simulink model "inverse_kinematics_calculator"  (R2019b)
settings: Solver=VariableStepAuto  StartTime=0.0  StopTime=4  RelTol=1e-3
libraries: simulink x3, robotcorelib x1, robotmaniplib x1
settings Model: Creator=PC  LastModifiedBy=PC

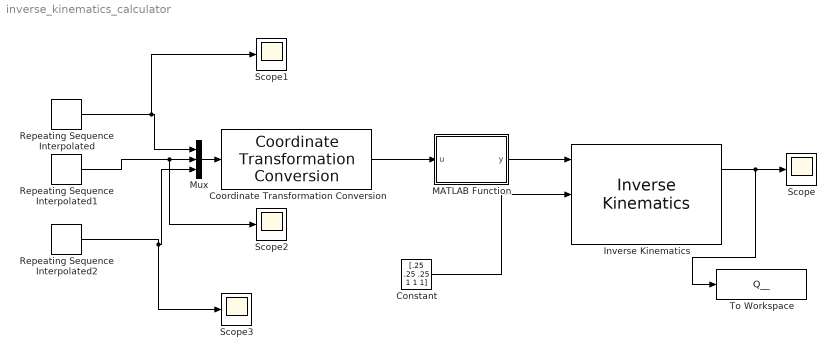
== system inverse_kinematics_calculator ==
  Constant : Constant  Value=[.25 .25 .25 1 1 1]
  Coordinate Transformation Conversion : robotcorelib/Coordinate Transformation Conversion  InputRepresentation=Translation Vector  InputEulerSequence=ZYX  ShowTrVecInputPort=on  OutputRepresentation=Homogeneous Transformation  OutputEulerSequence=ZYX  ShowTrVecOutputPort=on  SimulateUsing=Interpreted execution
      settings: SourceProductBaseCode=RO
  Inverse Kinematics : robotmaniplib/Inverse Kinematics  RigidBodyTree=robot  EndEffector=iiwa_link_ee_kuka  ShowInfo=on  SolverName=BFGS Gradient Projection  EnforceJointLimits=off  MaxIterations=1500  MaxTime=100  GradientTolerance=1e-7  SolutionTolerance=1e-6  StepTolerance=1e-14  ErrorChangeTolerance=1e-12  UseErrorDamping=on  DampingBias=0.0025  SimulateUsing=Interpreted execution
      settings: SourceProductName=Robotics System Toolbox
  MATLAB Function : MATLAB Function  TreatAsAtomicUnit=on
  Mux : Mux  Inputs=3
  Repeating Sequence Interpolated : simulink/Sources/Repeating Sequence Interpolated  OutValues=x  TimeValues=[0 1 2 3]  LookUpMeth=Interpolation-Use End Values  tsamp=1  OutMin=[]  OutMax=[]  OutDataTypeStr=double  OutputDataTypeScalingMode=double  OutDataType=fixdt(0,8)  OutScaling=2^-10
  Repeating Sequence Interpolated1 : simulink/Sources/Repeating Sequence Interpolated  OutValues=y  TimeValues=[0 1 2 3]  LookUpMeth=Interpolation-Use End Values  tsamp=1  OutMin=[]  OutMax=[]  OutDataTypeStr=double  OutputDataTypeScalingMode=double  OutDataType=fixdt(0,8)  OutScaling=2^-10
  Repeating Sequence Interpolated2 : simulink/Sources/Repeating Sequence Interpolated  OutValues=z  TimeValues=[0 1 2 3]  LookUpMeth=Interpolation-Use End Values  tsamp=1  OutMin=[]  OutMax=[]  OutDataTypeStr=double  OutputDataTypeScalingMode=double  OutDataType=fixdt(0,8)  OutScaling=2^-10
  Scope{,1..3} (4 alike) : Scope
  To Workspace : ToWorkspace  VariableName=Q__  SaveFormat=Timeseries  SampleTime=1
  wires:
  Repeating Sequence Interpolated/1 -> Scope1/1, Mux/1
  Repeating Sequence Interpolated1/1 -> Scope2/1, Mux/2
  Repeating Sequence Interpolated2/1 -> Scope3/1, Mux/3
  Mux/1 -> Coordinate Transformation Conversion/1
  Coordinate Transformation Conversion/1 -> MATLAB Function/1(u)
  Constant/1 -> Inverse Kinematics/2
  Inverse Kinematics/1 -> To Workspace/1, Scope/1
  MATLAB Function/1(y) -> Inverse Kinematics/1

== matlab function inverse_kinematics_calculator/MATLAB Function ==
  data: u input; y output
function y = fcn(u)
u(1:3,1:3) = [0 0 0; 0 0 0; 0 0 0];
u(1,3) = -1; 
u(2,2) = 1; 
u(3,1) = 1
y = u;
